simulink model "untitled"  (R2015a)
settings: Solver=ode45  StartTime=0.0  StopTime=1.8  RelTol=1e-3
values from neighbouring files (symbols this model uses):
  Gur = (p1*p2*p3*p4*s^2*(4*k*(jl+n^2*eta*(jm+jg+js))+4*d*(jl+n^2*eta*(jm+jg+js))*s+(2*jm+js)*(2*jl+n^2*eta*(2*jg+js))*s^2))/(kt*n*eta*k*(p1-s)*(p2-s)*(p3-s)*(p4-s))    [current_by_ref.m]
  Gurs = (p1*p2*p3*p4*s^2*4*(jl+n^2*eta*(jm+jg+js)))/(kt*n*eta*(p1-s)*(p2-s)*(p3-s)*(p4-s))    [current_by_ref.m]
libraries: simulink x2
settings Model: Creator=Goodman  LastModifiedBy=anqingd

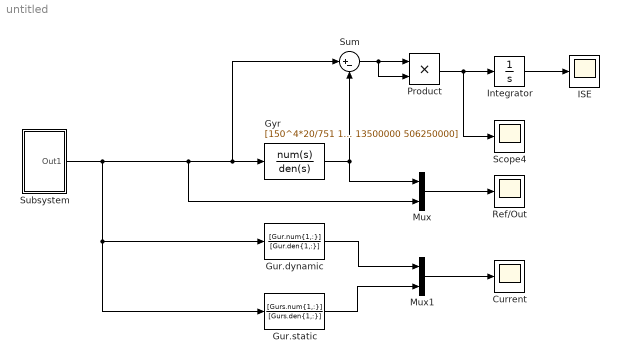
== system untitled ==
  Current : Scope
      settings: ShowLegends=on
  Gur.dynamic : TransferFcn  Numerator=[Gur.num{1,:}]  Denominator=[Gur.den{1,:}]
  Gur.static : TransferFcn  Numerator=[Gurs.num{1,:}]  Denominator=[Gurs.den{1,:}]
  Gyr : TransferFcn  Numerator=[150^4*20/751 150^4]  Denominator=[1 600 135000 13500000 506250000]
  ISE : Scope
  Integrator : Integrator
  Mux : Mux  Inputs=2
  Mux1 : Mux  Inputs=2
  Product : Product
  Ref/Out : Scope
      settings: SaveName=ScopeData3
  Scope4 : Scope
      settings: SaveName=ScopeData4
  Subsystem : Subsystem
  Sum : Sum  Inputs=|+-
  wires:
  Gyr/1 -> Mux/1, Sum/2
  Sum/1 -> Product/2, Product/1
  Product/1 -> Scope4/1, Integrator/1
  Integrator/1 -> ISE/1
  Mux/1 -> Ref/Out/1
  Subsystem/1(Out1) -> Gur.static/1, Gur.dynamic/1, Sum/1, Gyr/1, Mux/2
  Gur.dynamic/1 -> Mux1/1
  Mux1/1 -> Current/1
  Gur.static/1 -> Mux1/2

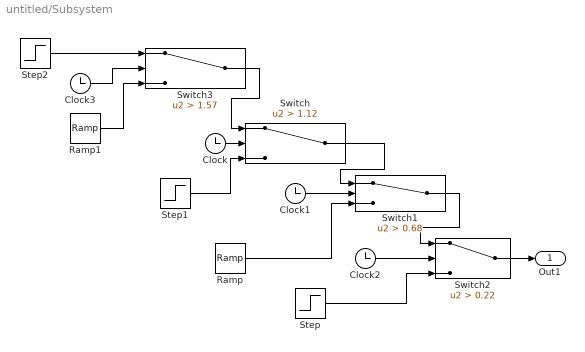
== system untitled/Subsystem ==
  Clock{,1..3} (4 alike) : Clock
  Ramp : simulink/Sources/Ramp  slope=3/0.46  start=0.22  X0=0
  Ramp1 : simulink/Sources/Ramp  slope=-3/0.45  start=1.12  X0=3
  Step : Step  Time=0  After=0  SampleTime=0
  Step1 : Step  Time=0  After=3  SampleTime=0
  Step2 : Step  Time=0  After=0  SampleTime=0
  Switch : Switch  Criteria=u2 > Threshold  Threshold=1.12
  Switch1 : Switch  Criteria=u2 > Threshold  Threshold=0.68
  Switch2 : Switch  Criteria=u2 > Threshold  Threshold=0.22
  Switch3 : Switch  Criteria=u2 > Threshold  Threshold=1.57
  Out1 : Outport
  wires:
  Ramp1/1 -> Switch3/3
  Switch/1 -> Switch1/1
  Step2/1 -> Switch3/1
  Switch1/1 -> Switch2/1
  Switch3/1 -> Switch/1
  Switch2/1 -> Out1/1
  Clock3/1 -> Switch3/2
  Ramp/1 -> Switch1/3
  Clock2/1 -> Switch2/2
  Step1/1 -> Switch/3
  Clock1/1 -> Switch1/2
  Step/1 -> Switch2/3
  Clock/1 -> Switch/2
